simulink library "SimscapeCustomComponents_lib"  (R2025b)
settings: Solver=VariableStepAuto  StartTime=0.0  StopTime=10.0  RelTol=1e-3
undefined symbols (not defined in the file or in its folder): base, baseVdc, capacity, DiscIntNeverNeededParam, ee_sli_rtmsupport, filterInductance, freqeuncy, frequency, gcbh, gflInverter, gfmInverter, iMaxPU, Inertia, initialSOC, plantRating, solar, Ts, ups, Vac, windSystem, windTurbine
libraries: fl_lib x397, nesl_utility x171, eeGeneralControl x85, ee_lib x82, simulink x72, datacenter_lib x68, eeTransforms x38, slpidlib x24, buildingEnergy_lib x20, SimscapeFluids_lib x17, eeSinusoidalMeasurementV2 x8, eePwmGenerator x8
(part 14 of 24)

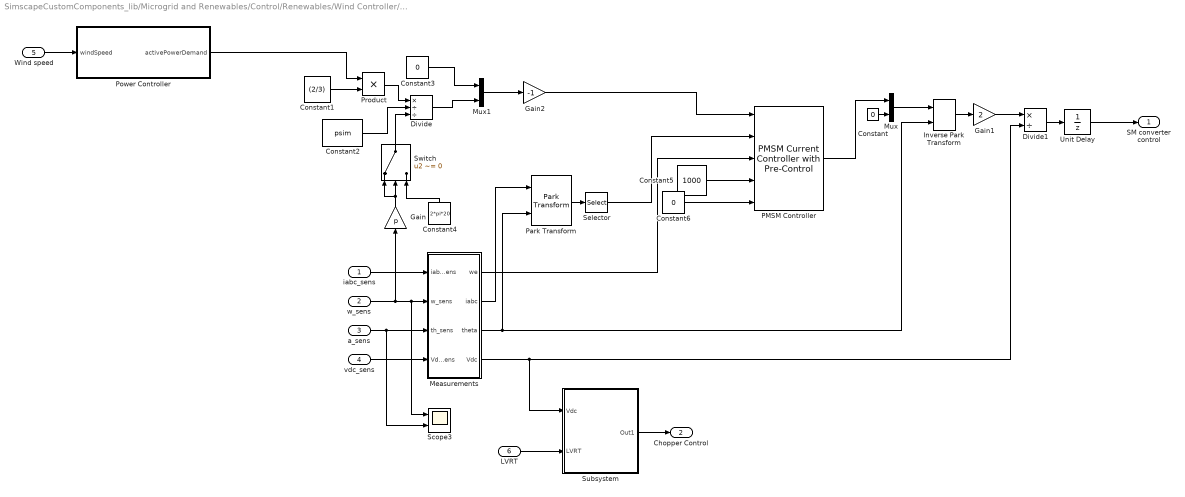
== system SimscapeCustomComponents_lib/Microgrid and Renewables/Control/Renewables/Wind Controller/Machine Converter Control ==
  iabc_sens : Inport
  w_sens : Inport  Port=2
  a_sens : Inport  Port=3
  vdc_sens : Inport  Port=4
  Wind speed : Inport  Port=5
  LVRT : Inport  Port=6
  Constant : Constant  Value=0  SampleTime=-1
  Constant1 : Constant  Value=(2/3)
  Constant2 : Constant  Value=psim
  Constant3 : Constant  Value=0
  Constant4 : Constant  Value=2*pi*20
  Constant5 : Constant  Value=1000  VectorParams1D=off  SampleTime=-1
  Constant6 : Constant  Value=0
  Divide : Product  Inputs=*//
  Divide1 : Product  Inputs=*/
  Gain : Gain  Gain=p
  Gain1 : Gain  Gain=2
  Gain2 : Gain  Gain=-1
  Inverse Park Transform : eeTransforms/Inverse Park Transform  AxisAlignment=Q-axis  PowerInvariant=off
  Measurements : Subsystem
  Mux : Mux  Inputs=2
  Mux1 : Mux  Inputs=2
  PMSM Controller : eePmsmCurrentController/PMSM Current Controller with Pre-Control  Kp_id=Kdip_sm  Ki_id=Kdii_sm  Kaw_id=0  Kp_iq=Kqip_sm  Ki_iq=Kqii_sm  Kaw_iq=0  Ts=-1  Tsd=0.001  AxisPrio=Q-axis  ActZC=off  ActFF=on  idVect=[-1, 0, 1]  iqVect=[-2000, 0, 2000]  LdMatrix=Ld* ones(3, 3)  LqMatrix=Lq* ones(3, 3)  psimMatrix=psim * ones(3, 3)
  Park Transform : eeTransforms/Park Transform  AxisAlignment=Q-axis  PowerInvariant=off
  Power Controller : Subsystem
  Product : Product
  Scope3 : Scope  NumInputPorts=2
      settings: ActiveDisplayYMinimum=-0.53154558960654574  ActiveDisplayYMaximum=3.2068078785969831  DataLoggingVariableName=ScopeData23
  Selector : Selector  InputPortWidth=3  IndexOptions=Index vector (dialog)  Indices=[1 2]  OutputSizes=1
  Subsystem : Subsystem
  Switch : Switch  Criteria=u2 ~= 0  SaturateOnIntegerOverflow=off  InputSameDT=off
  Unit Delay : UnitDelay  SampleTime=-1
  SM converter control : Outport  VectorParamsAs1DForOutWhenUnconnected=off
  Chopper Control : Outport  Port=2
  wires:
  Product/1 -> Divide/1
  Measurements/1(we) -> PMSM Controller/3
  Unit Delay/1 -> SM converter control/1
  Wind speed/1 -> Power Controller/1(windSpeed)
  Selector/1 -> PMSM Controller/2
  LVRT/1 -> Subsystem/2(LVRT)
  Divide/1 -> Mux1/2
  Constant4/1 -> Switch/3
  Gain1/1 -> Divide1/1
  PMSM Controller/1 -> Mux/1
  Mux1/1 -> Gain2/1
  Power Controller/1(activePowerDemand) -> Product/1
  Divide1/1 -> Unit Delay/1
  Constant2/1 -> Divide/2
  Constant1/1 -> Product/2
  Park Transform/1 -> Selector/1
  iabc_sens/1 -> Measurements/1(iabc_sens)
  Constant/1 -> Mux/2
  Measurements/2(iabc) -> Park Transform/1
  Constant6/1 -> PMSM Controller/5
  Switch/1 -> Divide/3
  Inverse Park Transform/1 -> Gain1/1
  Mux/1 -> Inverse Park Transform/1
  Gain2/1 -> PMSM Controller/1
  Measurements/4(Vdc) -> Subsystem/1(Vdc), Divide1/2
  vdc_sens/1 -> Measurements/4(Vdc_sens)
  Constant5/1 -> PMSM Controller/4
  Subsystem/1(Out1) -> Chopper Control/1
  Gain/1 -> Switch/1, Switch/2
  Constant3/1 -> Mux1/1
  a_sens/1 -> Scope3/2, Measurements/3(th_sens)
  w_sens/1 -> Gain/1, Scope3/1, Measurements/2(w_sens)
  Measurements/3(theta) -> Park Transform/2, Inverse Park Transform/2

== system SimscapeCustomComponents_lib/Microgrid and Renewables/Control/Renewables/Wind Controller/Wind Grid-side Converter Controller ==
  QRef : Inport
  BusElementIn : Inport  Port=2  PortName=VIBus  Element=Vmag
  BusElementIn4 : Inport  Port=2  PortName=VIBus  Element=Vmag
  BusElementIn1 : Inport  Port=2  PortName=VIBus  Element=Iabc
  BusElementIn2 : Inport  Port=2  PortName=VIBus  Element=Vq
  BusElementIn3 : Inport  Port=2  PortName=VIBus  Element=Vd
  BusElementIn5 : Inport  Port=2  PortName=VIBus  Element=Theta
  BusElementIn6 : Inport  Port=2  PortName=VIBus  Element=Theta
  LVRT : Inport  Port=3
  Vdc : Inport  Port=4
  Constant : Constant  Value=Vdc
  Current_controller : Subsystem
  "DC Bus Chopper control " : Subsystem
  DC voltage controller & current reference : Subsystem
  Demux : Demux  Outputs=3
  Inverse Park Transform1 : eeTransforms/Inverse Park Transform  AxisAlignment=Q-axis  PowerInvariant=off
  Park Transform1 : eeTransforms/Park Transform  AxisAlignment=Q-axis  PowerInvariant=off
  Terminator : Terminator
  Unit Delay2 : UnitDelay  SampleTime=Ts
  FRT : Outport
  m_abc : Outport  Port=2
  wires:
  BusElementIn3/1 -> Current_controller/5(Vd)
  BusElementIn1/1 -> Park Transform1/1
  DC voltage controller & current reference/2(iq_ref) -> Current_controller/4(iqref)
  DC voltage controller & current reference/1(id_ref) -> Current_controller/3(id-ref)
  Demux/2 -> Current_controller/2(iq)
  Demux/1 -> Current_controller/1(iWindd)
  Park Transform1/1 -> Demux/1
  BusElementIn2/1 -> Current_controller/6(Vq)
  Inverse Park Transform1/1 -> Unit Delay2/1
  Unit Delay2/1 -> m_abc/1
  Current_controller/1(Refrence_mdq0) -> Inverse Park Transform1/1
  BusElementIn6/1 -> Park Transform1/2
  BusElementIn5/1 -> Inverse Park Transform1/2
  BusElementIn4/1 -> DC voltage controller & current reference/2(Vmag)
  LVRT/1 -> DC voltage controller & current reference/5(lvrt.iq)
  QRef/1 -> DC voltage controller & current reference/1(Q_ref)
  BusElementIn/1 -> "DC Bus Chopper control "/1(In1)
  "DC Bus Chopper control "/1(Out1) -> FRT/1
  Demux/3 -> Terminator/1
  Vdc/1 -> DC voltage controller & current reference/3(Wind_Mpp_vdc)
  Constant/1 -> DC voltage controller & current reference/4(Wind_vdc)

== system SimscapeCustomComponents_lib/Microgrid and Renewables/Sources/Generator Integrated/Detailed/AVR and Exciter ==
  AVR : eeSmDC2C/SM DC2C  E_FD0=1.01  Ts=-1  R_C=0  X_C=0  T_R=0  K_A=300  T_A=0.06  T_B=0  T_C=0  K_F=0.058  T_F=0.62  V_Rmax=4.5  V_Rmin=-4.5  oelInputLocation=Unused  uelInputLocation=Unused  sclInputLocation=Unused  K_E=1  T_E=1.33  E_FDmin=-99  E_1=3.05  S_E_E1=0.279  E_2=2.29  S_E_E2=0.117
  Constant{3,5..9} (6 alike) : Constant  Value=0
  Constant4 : Constant  Value=1.05
  "E_FD Simulink-PS " : nesl_utility/Simulink-PS Converter  PhysicalDomain=network_engine_domain  SubClassName=ps_input  LeftPortType=input  RightPortType=output  PseudoPeriodic=off  Frequencies=[]  NoiseDistribution=none  NoiseParameters=[]  Unit=1  AffineConversion=off  FilteringAndDerivatives=provide  SimscapeFilterOrder=1  InputFilterTimeConstant=.001  UdotUserProvided=0
  Exciter : ee_lib/Electromechanical/Synchronous/Synchronous Machine Field Circuit  unit_option=ee.enum.unit.pu  SRated=genRating*1000 V*A  FRated=frequency Hz  fieldCircuitParameterization_option=ee.enum.sm.fieldparameterization.current  baseEfd=200 V  baseIfd=100 A  parameterization_option=2  Ladu=1.66  Rfd=0.0006  Xl=0.01  Xd=0.344  Xdd=0.026  Xddd=0.018  d_option=ee.enum.circuit.short  Td0d=machine.tauDAxisTransient s  Tdd=0.03 s  Td0dd=machine.tauDAxisSubTransient s  Tddd=0.008 s
      settings: InternalSimscapePortConfiguration="{\"Bottom\":[],\"Left\":[{\"id\":\"Efd_pu\",\"label\":\"Efd_pu\",\"type\":\"input\"},{\"id\":\"Ifd_pu\",\"label\":\"Ifd_pu\",\"type\":\"output\"}],\"Right\":[{\"id\":\"fd_p\",\"label\":\"fd+\",\"type\":\"foundation.electrical.electrical\"},{\"id\":\"fd_n\",\"label\":\"fd-\",\"type\":\"foundation.electrical.electrical\"}],\"Top\":[]}"
  I_FD PS-Simulink : nesl_utility/PS-Simulink Converter  PhysicalDomain=network_engine_domain  SubClassName=ps_output  LeftPortType=input  RightPortType=output  PseudoPeriodic=off  Frequencies=[]  VectorFormat=1-D array  Unit=1  AffineConversion=off
  Terminal Current Measurement : ee_lib/Electromechanical/Synchronous/Synchronous Machine Measurement  output_idx=15
      settings: InternalSimscapePortConfiguration="{\"Bottom\":[],\"Left\":[{\"id\":\"pu_input\",\"label\":\"pu\",\"type\":\"input\"}],\"Right\":[{\"id\":\"pu_output\",\"label\":\"o\",\"type\":\"output\"}],\"Top\":[]}"
  Terminal Current PS-Simulink : nesl_utility/PS-Simulink Converter  PhysicalDomain=network_engine_domain  SubClassName=ps_output  LeftPortType=input  RightPortType=output  PseudoPeriodic=off  Frequencies=[]  VectorFormat=1-D array  Unit=1  AffineConversion=off
  Terminal Voltage Measurement : ee_lib/Electromechanical/Synchronous/Synchronous Machine Measurement  output_idx=14
      settings: InternalSimscapePortConfiguration="{\"Bottom\":[],\"Left\":[{\"id\":\"pu_input\",\"label\":\"pu\",\"type\":\"input\"}],\"Right\":[{\"id\":\"pu_output\",\"label\":\"o\",\"type\":\"output\"}],\"Top\":[]}"
  Terminal Voltage PS-Simulink : nesl_utility/PS-Simulink Converter  PhysicalDomain=network_engine_domain  SubClassName=ps_output  LeftPortType=input  RightPortType=output  PseudoPeriodic=off  Frequencies=[]  VectorFormat=1-D array  Unit=1  AffineConversion=off
  Terminator : Terminator
  Unit Delay : UnitDelay  InitialCondition=1.32943  SampleTime=-1
  pu : PMIOPort  Side=Left
  fd+ : PMIOPort  Port=2  Side=Right
  fd- : PMIOPort  Port=3  Side=Right
  wires:
  Terminal Current PS-Simulink/1 -> AVR/4
  AVR/1 -> "E_FD Simulink-PS "/1
  Constant9/1 -> AVR/9
  Constant8/1 -> AVR/8
  Constant7/1 -> AVR/7
  Constant6/1 -> AVR/6
  Constant5/1 -> AVR/5
  Constant4/1 -> AVR/1
  Constant3/1 -> AVR/2
  Terminal Voltage PS-Simulink/1 -> AVR/3
  I_FD PS-Simulink/1 -> Unit Delay/1
  Unit Delay/1 -> Terminator/1
  connections:
  Terminal Current Measurement/RConn1 -- Terminal Current PS-Simulink/LConn1
  Terminal Voltage Measurement/RConn1 -- Terminal Voltage PS-Simulink/LConn1
  pu/RConn1 -- Terminal Current Measurement/LConn1 -- Terminal Voltage Measurement/LConn1
  Exciter/RConn1 -- fd+/RConn1
  fd-/RConn1 -- Exciter/RConn2
  I_FD PS-Simulink/LConn1 -- Exciter/LConn2
  "E_FD Simulink-PS "/RConn1 -- Exciter/LConn1

== system SimscapeCustomComponents_lib/Microgrid and Renewables/Sources/Generator Integrated/Detailed/Governor and Prime Mover  ==
  PRef : Inport
  Governor : Subsystem
  Ideal Torque Source : fl_lib/Mechanical/Mechanical Sources/Ideal Torque Source
  Mechanical Rotational Reference : fl_lib/Mechanical/Rotational Elements/Mechanical Rotational Reference
  Non-reheat turbine : Subsystem
  PS-Simulink Converter : nesl_utility/PS-Simulink Converter  PhysicalDomain=network_engine_domain  SubClassName=ps_output  LeftPortType=input  RightPortType=output  PseudoPeriodic=off  Frequencies=[]  VectorFormat=1-D array  Unit=1  AffineConversion=off
  Rotor Velocity Measurement : ee_lib/Electromechanical/Synchronous/Synchronous Machine Measurement  output_idx=4
      settings: InternalSimscapePortConfiguration="{\"Bottom\":[],\"Left\":[{\"id\":\"pu_input\",\"label\":\"pu\",\"type\":\"input\"}],\"Right\":[{\"id\":\"pu_output\",\"label\":\"o\",\"type\":\"output\"}],\"Top\":[]}"
  Scope : Scope
  Simulink-PS Converter : nesl_utility/Simulink-PS Converter  PhysicalDomain=network_engine_domain  SubClassName=ps_input  LeftPortType=input  RightPortType=output  PseudoPeriodic=off  Frequencies=[]  NoiseDistribution=none  NoiseParameters=[]  Unit=1  AffineConversion=off  FilteringAndDerivatives=zero  SimscapeFilterOrder=1  InputFilterTimeConstant=0.001  UdotUserProvided=1
  scale by base_torque : Gain  Gain=base_torque
  R : PMIOPort  Side=Right
  C : PMIOPort  Port=2  Side=Right
  pu : PMIOPort  Port=3  Side=Left
  wires:
  PS-Simulink Converter/1 -> Governor/1(pu_velocity)
  Governor/1(delta_y) -> Non-reheat turbine/1(delta_y)
  Non-reheat turbine/1(torque) -> Scope/1, scale by base_torque/1
  scale by base_torque/1 -> Simulink-PS Converter/1
  PRef/1 -> Governor/2(PRef)
  connections:
  C/RConn1 -- Ideal Torque Source/RConn2 -- Mechanical Rotational Reference/LConn1
  Ideal Torque Source/LConn1 -- R/RConn1
  pu/RConn1 -- Rotor Velocity Measurement/LConn1
  PS-Simulink Converter/LConn1 -- Rotor Velocity Measurement/RConn1
  Simulink-PS Converter/RConn1 -- Ideal Torque Source/RConn1

== system SimscapeCustomComponents_lib/Microgrid and Renewables/Sources/Generator Integrated/Detailed/Measurements ==
  Current and Voltage Sensor (Three-Phase) : ee_lib/Sensors & Transducers/Current and Voltage Sensor (Three-Phase)  vMeasurementType=ee.enum.vmeasurement.ll  outputUnit=ee.enum.unit.pu  SRated=genRating*1000 A*V  VRated=Vac V  I_specify=off  I_priority=None  I=[0, 0, 0] A  I_nominal_specify=off  I_nominal_value=1  I_nominal_unit=A  V_specify=off  V_priority=None  V=[0, 0, 0] V  V_nominal_specify=off  V_nominal_value=1  V_nominal_unit=V
      settings: InternalSimscapePortConfiguration="{\"Bottom\":[],\"Left\":[{\"id\":\"N1\",\"label\":\"~1\",\"type\":\"foundation.electrical.three_phase\"}],\"Right\":[{\"id\":\"V_output\",\"label\":\"V\",\"type\":\"output\"},{\"id\":\"I_output\",\"label\":\"I\",\"type\":\"output\"},{\"id\":\"N2\",\"label\":\"~2\",\"type\":\"foundation.electrical.three_phase\"}],\"Top\":[]}"
  Gain : Gain  Gain=1/(genRating*1000)
  Gain1 : Gain  Gain=1/(genRating*1000)
  Low-Pass Filter (Discrete or Continuous)1 : eeGeneralControl/Low-Pass Filter (Discrete or Continuous)  K=1  T=0.1  B=inf  A=-inf  init_option=Inherited from block input  x0=0  Ts=-1
  Low-Pass Filter (Discrete or Continuous)2 : eeGeneralControl/Low-Pass Filter (Discrete or Continuous)  K=1  T=0.1  B=inf  A=-inf  init_option=Inherited from block input  x0=0  Ts=-1
  PS-Simulink Converter{,1..3} (4 alike) : nesl_utility/PS-Simulink Converter  PhysicalDomain=network_engine_domain  SubClassName=ps_output  LeftPortType=input  RightPortType=output  PseudoPeriodic=off  Frequencies=[]  VectorFormat=inherit  Unit=inherit  AffineConversion=off
  Power Sensor (Three-Phase) : ee_lib/Sensors & Transducers/Power Sensor (Three-Phase)  load_type=ee.enum.passive.type_balanced.balanced  f0=60 Hz
      settings: InternalSimscapePortConfiguration="{\"Bottom\":[],\"Left\":[{\"id\":\"N1\",\"label\":\"~1\",\"type\":\"foundation.electrical.three_phase\"}],\"Right\":[{\"id\":\"N2\",\"label\":\"~2\",\"type\":\"foundation.electrical.three_phase\"}],\"Top\":[{\"id\":\"Pm\",\"label\":\"P\",\"type\":\"output\"},{\"id\":\"Qm\",\"label\":\"Q\",\"type\":\"output\"}]}"
  In : PMIOPort  Side=Left
  ~ : PMIOPort  Port=2  Side=Right
  P : Outport
  Q : Outport  Port=2
  V : Outport  Port=3
  I : Outport  Port=4
  wires:
  PS-Simulink Converter/1 -> Low-Pass Filter (Discrete or Continuous)1/1
  PS-Simulink Converter1/1 -> Low-Pass Filter (Discrete or Continuous)2/1
  Low-Pass Filter (Discrete or Continuous)1/1 -> Gain/1
  Low-Pass Filter (Discrete or Continuous)2/1 -> Gain1/1
  PS-Simulink Converter2/1 -> V/1
  PS-Simulink Converter3/1 -> I/1
  Gain/1 -> P/1
  Gain1/1 -> Q/1
  connections:
  Current and Voltage Sensor (Three-Phase)/RConn1 -- PS-Simulink Converter2/LConn1
  PS-Simulink Converter/LConn1 -- Power Sensor (Three-Phase)/LConn2
  In/RConn1 -- Power Sensor (Three-Phase)/LConn1
  Current and Voltage Sensor (Three-Phase)/RConn3 -- ~/RConn1
  PS-Simulink Converter1/LConn1 -- Power Sensor (Three-Phase)/LConn3
  Current and Voltage Sensor (Three-Phase)/LConn1 -- Power Sensor (Three-Phase)/RConn1
  Current and Voltage Sensor (Three-Phase)/RConn2 -- PS-Simulink Converter3/LConn1

== system SimscapeCustomComponents_lib/Microgrid and Renewables/Sources/Generator Integrated/Simplified/Exciter ==
  Current Sensor : fl_lib/Electrical/Electrical Sensors/Current Sensor
  Voltage Source : ee_lib/Sources/Voltage Source  dc_voltage=150 V  ac_voltage=0 V  ac_shift=0 rad  ac_frequency=frequency Hz  noise_mode=ee.enum.sources.noise.Disabled  PSD=0 V^2/Hz  sample_time=1e-3 s  repeatability=ee.enum.sources.repeatability.NotRepeatable  user_seed=0  auto_seed=3890346746  i_specify=off  i_priority=None  i=0 A  i_nominal_specify=off  i_nominal_value=1  i_nominal_unit=A  v_specify=off  v_priority=None  v=0 V  v_nominal_specify=off  v_nominal_value=1  v_nominal_unit=V
  + : PMIOPort  Side=Right
  - : PMIOPort  Port=2  Side=Right
  connections:
  Voltage Source/RConn1 -- -/RConn1
  Current Sensor/RConn2 -- +/RConn1
  Voltage Source/LConn1 -- Current Sensor/LConn1

== system SimscapeCustomComponents_lib/Microgrid and Renewables/Sources/Generator Integrated/Simplified/Measurements ==
  Current and Voltage Sensor (Three-Phase) : ee_lib/Sensors & Transducers/Current and Voltage Sensor (Three-Phase)  vMeasurementType=ee.enum.vmeasurement.ll  outputUnit=ee.enum.unit.pu  SRated=genRating*1000 A*V  VRated=Vac V  I_specify=off  I_priority=None  I=[0, 0, 0] A  I_nominal_specify=off  I_nominal_value=1  I_nominal_unit=A  V_specify=off  V_priority=None  V=[0, 0, 0] V  V_nominal_specify=off  V_nominal_value=1  V_nominal_unit=V
      settings: InternalSimscapePortConfiguration="{\"Bottom\":[],\"Left\":[{\"id\":\"N1\",\"label\":\"~1\",\"type\":\"foundation.electrical.three_phase\"}],\"Right\":[{\"id\":\"V_output\",\"label\":\"V\",\"type\":\"output\"},{\"id\":\"I_output\",\"label\":\"I\",\"type\":\"output\"},{\"id\":\"N2\",\"label\":\"~2\",\"type\":\"foundation.electrical.three_phase\"}],\"Top\":[]}"
  Gain : Gain  Gain=1/(genRating*1000)
  Gain1 : Gain  Gain=1/(genRating*1000)
  Low-Pass Filter (Discrete or Continuous)1 : eeGeneralControl/Low-Pass Filter (Discrete or Continuous)  K=1  T=0.1  B=inf  A=-inf  init_option=Inherited from block input  x0=0  Ts=-1
  Low-Pass Filter (Discrete or Continuous)2 : eeGeneralControl/Low-Pass Filter (Discrete or Continuous)  K=1  T=0.1  B=inf  A=-inf  init_option=Inherited from block input  x0=0  Ts=-1
  PS-Simulink Converter{,1..3} (4 alike) : nesl_utility/PS-Simulink Converter  PhysicalDomain=network_engine_domain  SubClassName=ps_output  LeftPortType=input  RightPortType=output  PseudoPeriodic=off  Frequencies=[]  VectorFormat=inherit  Unit=inherit  AffineConversion=off
  Power Sensor (Three-Phase) : ee_lib/Sensors & Transducers/Power Sensor (Three-Phase)  load_type=ee.enum.passive.type_balanced.balanced  f0=60 Hz
      settings: InternalSimscapePortConfiguration="{\"Bottom\":[],\"Left\":[{\"id\":\"N1\",\"label\":\"~1\",\"type\":\"foundation.electrical.three_phase\"}],\"Right\":[{\"id\":\"N2\",\"label\":\"~2\",\"type\":\"foundation.electrical.three_phase\"}],\"Top\":[{\"id\":\"Pm\",\"label\":\"P\",\"type\":\"output\"},{\"id\":\"Qm\",\"label\":\"Q\",\"type\":\"output\"}]}"
  In : PMIOPort  Side=Left
  ~ : PMIOPort  Port=2  Side=Right
  P : Outport
  Q : Outport  Port=2
  V : Outport  Port=3
  I : Outport  Port=4
  wires:
  PS-Simulink Converter/1 -> Low-Pass Filter (Discrete or Continuous)1/1
  PS-Simulink Converter1/1 -> Low-Pass Filter (Discrete or Continuous)2/1
  Low-Pass Filter (Discrete or Continuous)1/1 -> Gain/1
  Low-Pass Filter (Discrete or Continuous)2/1 -> Gain1/1
  PS-Simulink Converter2/1 -> V/1
  PS-Simulink Converter3/1 -> I/1
  Gain/1 -> P/1
  Gain1/1 -> Q/1
  connections:
  Current and Voltage Sensor (Three-Phase)/RConn1 -- PS-Simulink Converter2/LConn1
  PS-Simulink Converter/LConn1 -- Power Sensor (Three-Phase)/LConn2
  In/RConn1 -- Power Sensor (Three-Phase)/LConn1
  Current and Voltage Sensor (Three-Phase)/RConn3 -- ~/RConn1
  PS-Simulink Converter1/LConn1 -- Power Sensor (Three-Phase)/LConn3
  Current and Voltage Sensor (Three-Phase)/LConn1 -- Power Sensor (Three-Phase)/RConn1
  Current and Voltage Sensor (Three-Phase)/RConn2 -- PS-Simulink Converter3/LConn1

== system SimscapeCustomComponents_lib/Microgrid and Renewables/Sources/Generator Integrated/Simplified/Prime Mover ==
  PRef : Inport
  Ideal Torque Source : fl_lib/Mechanical/Mechanical Sources/Ideal Torque Source
  Mechanical Rotational Reference : fl_lib/Mechanical/Rotational Elements/Mechanical Rotational Reference
  Saturation : Saturate  UpperLimit=1  LowerLimit=0
  Scope : Scope
      settings: ActiveDisplayYMinimum=-1.25  ActiveDisplayYMaximum=1.25
  Simulink-PS Converter : nesl_utility/Simulink-PS Converter  PhysicalDomain=network_engine_domain  SubClassName=ps_input  LeftPortType=input  RightPortType=output  PseudoPeriodic=off  Frequencies=[]  NoiseDistribution=none  NoiseParameters=[]  Unit=1  AffineConversion=off  FilteringAndDerivatives=zero  SimscapeFilterOrder=1  InputFilterTimeConstant=0.001  UdotUserProvided=1
  scale by base_torque : Gain  Gain=genRating*1000/(2*pi*frequency)
  R : PMIOPort  Side=Right
  C : PMIOPort  Port=2  Side=Right
  wires:
  PRef/1 -> Saturation/1, Scope/1
  scale by base_torque/1 -> Simulink-PS Converter/1
  Saturation/1 -> scale by base_torque/1
  connections:
  Ideal Torque Source/LConn1 -- R/RConn1
  C/RConn1 -- Mechanical Rotational Reference/LConn1 -- Ideal Torque Source/RConn2
  Simulink-PS Converter/RConn1 -- Ideal Torque Source/RConn1

== system SimscapeCustomComponents_lib/Microgrid and Renewables/Sources/Solar Plant/Converter/Average ==
  mabc : Inport
  Converter : ee_lib/Semiconductors & Converters/Converters/Average-Value Voltage Source Converter (Three-Phase)  port_option=ee.enum.threePhasePort.composite  frequency_option=ee.enum.converters.frequency.variable  input_option=ee.enum.converters.inputOption.ModWave  FRated=60 Hz  losses_parameterization=ee.enum.converters.losses.fixed  Pfixed=0.5 W  ks=0.01  kc1=1.7 V  kc2=0.01 Ohm  Ploss_vect=[100, 800, 1870, 3250, 4900] W  Irms_vect=[10, 100, 200, 300, 400] A  Vdc_nom=300 V  thermal_mass=30000 J/K  temperature_specify=off  temperature_priority=High  temperature=298.15 K  temperature_nominal_specify=off  temperature_nominal_value=1  temperature_nominal_unit=K
      settings: InternalSimscapePortConfiguration="{\"Bottom\":[],\"Left\":[{\"id\":\"ModWave\",\"label\":\"ModWave\",\"type\":\"input\"},{\"id\":\"N\",\"label\":\"~\",\"type\":\"foundation.electrical.three_phase\"}],\"Right\":[{\"id\":\"p\",\"label\":\"+\",\"type\":\"foundation.electrical.electrical\"},{\"id\":\"n\",\"label\":\"-\",\"type\":\"foundation.electrical.electrical\"}],\"Top\":[]}"
  Simulink-PS Converter : nesl_utility/Simulink-PS Converter  PhysicalDomain=network_engine_domain  SubClassName=ps_input  LeftPortType=input  RightPortType=output  PseudoPeriodic=off  Frequencies=[]  NoiseDistribution=none  NoiseParameters=[]  Unit=1  AffineConversion=off  FilteringAndDerivatives=provide  SimscapeFilterOrder=1  InputFilterTimeConstant=0.001  UdotUserProvided=0
  + : PMIOPort  Side=Left
  - : PMIOPort  Port=2  Side=Left
  ~ : PMIOPort  Port=3  Side=Right
  wires:
  mabc/1 -> Simulink-PS Converter/1
  connections:
  +/RConn1 -- Converter/RConn1
  -/RConn1 -- Converter/RConn2
  ~/RConn1 -- Converter/LConn2
  Simulink-PS Converter/RConn1 -- Converter/LConn1

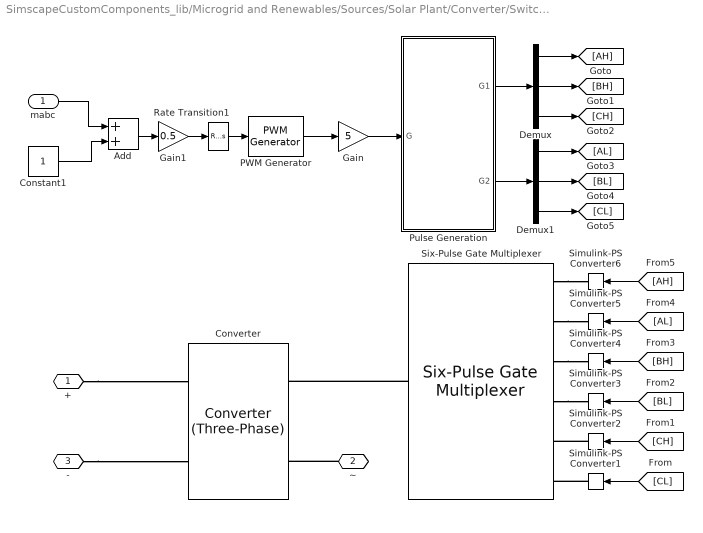
== system SimscapeCustomComponents_lib/Microgrid and Renewables/Sources/Solar Plant/Converter/Switching ==
  mabc : Inport
  Add : Sum
  Constant1 : Constant
  Converter : ee_lib/Semiconductors & Converters/Converters/Converter (Three-Phase)  port_option=ee.enum.threePhasePort.composite  fidelity_option=ee.enum.converters.fidelity.detailed  device_type=ee.enum.converters.switchingdevice.ideal  showThermalPort=false  K=0  Vth=1 V  Vgt=1 V  Vgt_off=-1 V  Ih=1 A  Vf=0.8 V  Ron=0.001 Ohm  Rds=0.001 Ohm  Goff=1e-6 1/Ohm  Eon_scalar=22.86e-3 J  Eoff_scalar=17.14e-3 J  Eoff_natural_commutation=10e-3 J  Voff=300 V  Iout_scalar=600 A  onCurrentMeasDelay=0 s  useCurrentFromPreviousCycle=false  useVoltageFromPreviousCycle=false  diode_param=ee.enum.converters.protectiondiode.nodynamics  diode_Vf=0.01 V  diode_Ron=0.0001 Ohm  diode_Goff=1e-5 1/Ohm  diode_C=50 nF  diode_iRM=-235 A  diode_iF=300 A  diode_idot=-50 A/us  diode_trr_param=ee.enum.converters.diodetrr.trr_factor  diode_trr_factor=3  diode_trr=15 us  diode_Qrr=1500 s*uA  diode_rec_loss_model=ee.enum.diode.reverseRecoveryModel.fixed  diode_ErecVal=0 J  diode_scaleWithIandV=false  diode_ErecMat=zeros(2, 3) J  diode_TjrecVec=[298.15, 398.15] K  diode_IfrecVec=[.1, 1, 10] A  diode_IrecVal=10 A  diode_VrecVal=10 V  diode_tFilter=1 / 1000 / 100 s  thermal_network_parameterization=ee.enum.thermalNetworkTopology.external  Rth=[.08, .5] K/W  Rth_Cauer=[.08, .1, .5] K/W  Rth_Foster=[.08, .14, .22, .16] K/W  thermal_mass_parameterization=ee.enum.thermalNetwork.timeconstant  thermal_mass=[.01, .5] J/K  thermal_mass_Cauer=[.01, .1, .5] J/K  thermal_mass_Foster=[.001, .005, .05, .5] J/K  thermal_time_constant=[.001, .2] s  thermal_time_constant_Cauer=[.001, .1, .2] s  thermal_time_constant_Foster=[7e-05, .0007, .01, .08] s  thermal_mass_initial_temperatures=[25, 25] degC  thermal_mass_initial_temperatures_Cauer=[25, 25, 25] degC  junction_thermal_mass=0.01 J/K  Tvec_initial_Foster=[25, 25, 25, 25] degC  snubber_type=ee.enum.converters.snubber.exclude  Cs=1e-7 F  Rs=0.1 Ohm  Vce_loss=[0, 150, 300] V
  Demux : Demux  Outputs=3
  Demux1 : Demux  Outputs=3
  Gain : Gain  Gain=5
  Gain1 : Gain  Gain=0.5
  PWM Generator : eePwmGenerator/PWM Generator  CarrCount=Up  Tper=1/(fSw*1000)  Tdelay=0  Ts=1/(10*fSw*1000)
  Pulse Generation : Subsystem
  Rate Transition1 : RateTransition  OutPortSampleTime=1/(10*fSw*1000)
  Simulink-PS Converter{1..6} (6 alike) : nesl_utility/Simulink-PS Converter  PhysicalDomain=network_engine_domain  SubClassName=ps_input  LeftPortType=input  RightPortType=output  PseudoPeriodic=off  Frequencies=[]  NoiseDistribution=none  NoiseParameters=[]  Unit=1  AffineConversion=off  FilteringAndDerivatives=provide  SimscapeFilterOrder=1  InputFilterTimeConstant=0.001  UdotUserProvided=0
  Six-Pulse Gate Multiplexer : ee_lib/Semiconductors & Converters/Converters/Six-Pulse Gate Multiplexer  port_option=ee.enum.controlport.ps
  + : PMIOPort  Side=Left
  ~ : PMIOPort  Port=2  Side=Right
  - : PMIOPort  Port=3  Side=Left
  wires:
  [BH] -> Simulink-PS Converter4/1
  Pulse Generation/1(G1) -> Demux/1
  Pulse Generation/2(G2) -> Demux1/1
  Rate Transition1/1 -> PWM Generator/1
  Demux/1 -> [AH]
  Demux1/2 -> [BL]
  [AL] -> Simulink-PS Converter5/1
  [CH] -> Simulink-PS Converter2/1
  mabc/1 -> Add/1
  PWM Generator/1 -> Gain/1
  Gain/1 -> Pulse Generation/1(G)
  Add/1 -> Gain1/1
  Constant1/1 -> Add/2
  [CL] -> Simulink-PS Converter1/1
  Demux/2 -> [BH]
  Demux/3 -> [CH]
  Gain1/1 -> Rate Transition1/1
  Demux1/3 -> [CL]
  [AH] -> Simulink-PS Converter6/1
  [BL] -> Simulink-PS Converter3/1
  Demux1/1 -> [AL]
  connections:
  -/RConn1 -- Converter/RConn2
  +/RConn1 -- Converter/RConn1
  Six-Pulse Gate Multiplexer/LConn4 -- Simulink-PS Converter3/RConn1
  Six-Pulse Gate Multiplexer/LConn1 -- Simulink-PS Converter6/RConn1
  Six-Pulse Gate Multiplexer/RConn1 -- Converter/LConn1
  Six-Pulse Gate Multiplexer/LConn3 -- Simulink-PS Converter4/RConn1
  Simulink-PS Converter1/RConn1 -- Six-Pulse Gate Multiplexer/LConn6
  Simulink-PS Converter2/RConn1 -- Six-Pulse Gate Multiplexer/LConn5
  Six-Pulse Gate Multiplexer/LConn2 -- Simulink-PS Converter5/RConn1
  ~/RConn1 -- Converter/LConn2

== system SimscapeCustomComponents_lib/Microgrid and Renewables/Sources/Solar Plant Integrated/Detailed/Measurements ==
  Current and Voltage Sensor (Three-Phase) : ee_lib/Sensors & Transducers/Current and Voltage Sensor (Three-Phase)  vMeasurementType=ee.enum.vmeasurement.lg  outputUnit=ee.enum.unit.pu  SRated=plantRating*1000 A*V  VRated=Vac V  I_specify=off  I_priority=None  I=[0, 0, 0] A  I_nominal_specify=off  I_nominal_value=1  I_nominal_unit=A  V_specify=off  V_priority=None  V=[0, 0, 0] V  V_nominal_specify=off  V_nominal_value=1  V_nominal_unit=V
      settings: InternalSimscapePortConfiguration="{\"Bottom\":[],\"Left\":[{\"id\":\"N1\",\"label\":\"~1\",\"type\":\"foundation.electrical.three_phase\"}],\"Right\":[{\"id\":\"V_output\",\"label\":\"V\",\"type\":\"output\"},{\"id\":\"I_output\",\"label\":\"I\",\"type\":\"output\"},{\"id\":\"N2\",\"label\":\"~2\",\"type\":\"foundation.electrical.three_phase\"}],\"Top\":[]}"
  Gain : Gain  Gain=1/(plantRating*1000)
  Gain1 : Gain  Gain=1/(plantRating*1000)
  Low-Pass Filter (Discrete or Continuous)1 : eeGeneralControl/Low-Pass Filter (Discrete or Continuous)  K=1  T=0.1  B=inf  A=-inf  init_option=Inherited from block input  x0=0  Ts=-1
  Low-Pass Filter (Discrete or Continuous)2 : eeGeneralControl/Low-Pass Filter (Discrete or Continuous)  K=1  T=0.1  B=inf  A=-inf  init_option=Inherited from block input  x0=0  Ts=-1
  PS-Simulink Converter{,1..3} (4 alike) : nesl_utility/PS-Simulink Converter  PhysicalDomain=network_engine_domain  SubClassName=ps_output  LeftPortType=input  RightPortType=output  PseudoPeriodic=off  Frequencies=[]  VectorFormat=inherit  Unit=inherit  AffineConversion=off
  Power Sensor (Three-Phase) : ee_lib/Sensors & Transducers/Power Sensor (Three-Phase)  load_type=ee.enum.passive.type_balanced.balanced  f0=60 Hz
      settings: InternalSimscapePortConfiguration="{\"Bottom\":[],\"Left\":[{\"id\":\"N1\",\"label\":\"~1\",\"type\":\"foundation.electrical.three_phase\"}],\"Right\":[{\"id\":\"N2\",\"label\":\"~2\",\"type\":\"foundation.electrical.three_phase\"}],\"Top\":[{\"id\":\"Pm\",\"label\":\"P\",\"type\":\"output\"},{\"id\":\"Qm\",\"label\":\"Q\",\"type\":\"output\"}]}"
  In : PMIOPort  Side=Left
  ~ : PMIOPort  Port=2  Side=Right
  P : Outport
  Q : Outport  Port=2
  V : Outport  Port=3
  I : Outport  Port=4
  wires:
  PS-Simulink Converter/1 -> Low-Pass Filter (Discrete or Continuous)1/1
  PS-Simulink Converter1/1 -> Low-Pass Filter (Discrete or Continuous)2/1
  Low-Pass Filter (Discrete or Continuous)1/1 -> Gain/1
  Low-Pass Filter (Discrete or Continuous)2/1 -> Gain1/1
  PS-Simulink Converter2/1 -> V/1
  PS-Simulink Converter3/1 -> I/1
  Gain/1 -> P/1
  Gain1/1 -> Q/1
  connections:
  Current and Voltage Sensor (Three-Phase)/RConn1 -- PS-Simulink Converter2/LConn1
  PS-Simulink Converter/LConn1 -- Power Sensor (Three-Phase)/LConn2
  In/RConn1 -- Power Sensor (Three-Phase)/LConn1
  Current and Voltage Sensor (Three-Phase)/RConn3 -- ~/RConn1
  PS-Simulink Converter1/LConn1 -- Power Sensor (Three-Phase)/LConn3
  Current and Voltage Sensor (Three-Phase)/LConn1 -- Power Sensor (Three-Phase)/RConn1
  Current and Voltage Sensor (Three-Phase)/RConn2 -- PS-Simulink Converter3/LConn1

== system SimscapeCustomComponents_lib/Microgrid and Renewables/Sources/Solar Plant Integrated/Detailed/PV Plant & Controller ==
  note: Plant
  note: Controller
  Insolation : Inport
  Pref : Inport  Port=2
  Qref : Inport  Port=3
  Vabc : Inport  Port=4
  Iabc : Inport  Port=5
  Mode : Inport  Port=6
  Controller : Subsystem
  Delay : Delay  DelayLength=1
  PV Plant : Subsystem  InitFcn=%solar.mask.restoreSolarLink(gcb);  mask(Solar Plant){capDC=capacitance, converterFidelity=Switching, fSw=fSw, ratedVoltage=Vac, nSeries=nSeries, nParallel=nParallel}
      mask prompts: capDC "DC bus capacitance (F)"; converterFidelity "Converter Fidelity"; fSw "Switching Frequency (kHz)"; ratedVoltage "Rated voltage on AC side (V)"; nSeries "Number of panels in series"; nParallel "Number of panels in parallel"
      mask help: This block represents the physical interface between the solar panels and the power converter. It models the electrical and dynamic characteristics of the solar panels connected to a converter, while expecting an external control signal for operation
      settings: CopyFcn=set_param(gcbh,'LinkStatus','none');  PreSaveFcn=%solar.mask.restoreSolarLink(gcb);  CloseFcn=%solar.mask.restoreSolarLink(gcb);
      mask TypeOptions converterFidelity: Converter/converterFidelity
      mask Callback converterFidelity: component.mask.converterFidelityPlant;
      mask TypeOptions fSw: Converter/fSw
      mask DialogControl Container4 Prompt: General
      mask DialogControl editSolarCell Prompt: Edit Solar Cell Parameters
      mask DialogControl editSolarCell Callback:
      | blockPath = [gcb,'/','PV Array'];
      | component.mask.openBlock(blockPath);;
      mask DialogControl editConverter Prompt: Edit converter parameters
      mask DialogControl editConverter Callback:
      | converterFidelity = get_param(gcb,'converterFidelity');
      | blockPath = [gcb,'/','Converter','/',converterFidelity,'/','Converter'];
      | component.mask.openBlock(blockPath);
      mask Display: image('solar1.png');
  Scope1 : Scope
      settings: ActiveDisplayYMinimum=-2.35685  ActiveDisplayYMaximum=2.29234  DataLoggingVariableName=ScopeData4
  Sensor Dynamics : Subsystem
  Simulink-PS Converter : nesl_utility/Simulink-PS Converter  PhysicalDomain=network_engine_domain  SubClassName=ps_input  LeftPortType=input  RightPortType=output  PseudoPeriodic=off  Frequencies=[]  NoiseDistribution=none  NoiseParameters=[]  Unit=1  AffineConversion=off  FilteringAndDerivatives=provide  SimscapeFilterOrder=1  InputFilterTimeConstant=0.001  UdotUserProvided=0
  abc : PMIOPort  Side=Right
  wires:
  Mode/1 -> Controller/7(Mode)
  Iabc/1 -> Controller/5(Iabc)
  Vabc/1 -> Controller/4(Vabc)
  Pref/1 -> Controller/6(Pref)
  Qref/1 -> Controller/1(Qref)
  Sensor Dynamics/1(I) -> Controller/2(ipv (A))
  Sensor Dynamics/2(V) -> Controller/3(vdc (V))
  Controller/1(vabcRef (pu)) -> Delay/1, Scope1/1
  Insolation/1 -> Simulink-PS Converter/1
  Delay/1 -> PV Plant/1(mabc)
  PV Plant/1(I) -> Sensor Dynamics/1(Iin)
  PV Plant/2(V) -> Sensor Dynamics/2(Vin)
  connections:
  PV Plant/LConn1 -- Simulink-PS Converter/RConn1
  abc/RConn1 -- PV Plant/RConn1

== system SimscapeCustomComponents_lib/Microgrid and Renewables/Sources/Solar Plant Integrated/Simplified/Measurements ==
  Current and Voltage Sensor (Three-Phase) : ee_lib/Sensors & Transducers/Current and Voltage Sensor (Three-Phase)  vMeasurementType=ee.enum.vmeasurement.lg  outputUnit=ee.enum.unit.pu  SRated=plantRating*1000 A*V  VRated=Vac V  I_specify=off  I_priority=None  I=[0, 0, 0] A  I_nominal_specify=off  I_nominal_value=1  I_nominal_unit=A  V_specify=off  V_priority=None  V=[0, 0, 0] V  V_nominal_specify=off  V_nominal_value=1  V_nominal_unit=V
      settings: InternalSimscapePortConfiguration="{\"Bottom\":[],\"Left\":[{\"id\":\"N1\",\"label\":\"~1\",\"type\":\"foundation.electrical.three_phase\"}],\"Right\":[{\"id\":\"V_output\",\"label\":\"V\",\"type\":\"output\"},{\"id\":\"I_output\",\"label\":\"I\",\"type\":\"output\"},{\"id\":\"N2\",\"label\":\"~2\",\"type\":\"foundation.electrical.three_phase\"}],\"Top\":[]}"
  Gain : Gain  Gain=1/(plantRating*1000)
  Gain1 : Gain  Gain=1/(plantRating*1000)
  Low-Pass Filter (Discrete or Continuous)1 : eeGeneralControl/Low-Pass Filter (Discrete or Continuous)  K=1  T=0.1  B=inf  A=-inf  init_option=Inherited from block input  x0=0  Ts=-1
  Low-Pass Filter (Discrete or Continuous)2 : eeGeneralControl/Low-Pass Filter (Discrete or Continuous)  K=1  T=0.1  B=inf  A=-inf  init_option=Inherited from block input  x0=0  Ts=-1
  PS-Simulink Converter{,1..3} (4 alike) : nesl_utility/PS-Simulink Converter  PhysicalDomain=network_engine_domain  SubClassName=ps_output  LeftPortType=input  RightPortType=output  PseudoPeriodic=off  Frequencies=[]  VectorFormat=inherit  Unit=inherit  AffineConversion=off
  Power Sensor (Three-Phase) : ee_lib/Sensors & Transducers/Power Sensor (Three-Phase)  load_type=ee.enum.passive.type_balanced.balanced  f0=60 Hz
      settings: InternalSimscapePortConfiguration="{\"Bottom\":[],\"Left\":[{\"id\":\"N1\",\"label\":\"~1\",\"type\":\"foundation.electrical.three_phase\"}],\"Right\":[{\"id\":\"N2\",\"label\":\"~2\",\"type\":\"foundation.electrical.three_phase\"}],\"Top\":[{\"id\":\"Pm\",\"label\":\"P\",\"type\":\"output\"},{\"id\":\"Qm\",\"label\":\"Q\",\"type\":\"output\"}]}"
  In : PMIOPort  Side=Left
  ~ : PMIOPort  Port=2  Side=Right
  P : Outport
  Q : Outport  Port=2
  V : Outport  Port=3
  I : Outport  Port=4
  wires:
  PS-Simulink Converter/1 -> Low-Pass Filter (Discrete or Continuous)1/1
  PS-Simulink Converter1/1 -> Low-Pass Filter (Discrete or Continuous)2/1
  Low-Pass Filter (Discrete or Continuous)1/1 -> Gain/1
  Low-Pass Filter (Discrete or Continuous)2/1 -> Gain1/1
  PS-Simulink Converter2/1 -> V/1
  PS-Simulink Converter3/1 -> I/1
  Gain/1 -> P/1
  Gain1/1 -> Q/1
  connections:
  Current and Voltage Sensor (Three-Phase)/RConn1 -- PS-Simulink Converter2/LConn1
  PS-Simulink Converter/LConn1 -- Power Sensor (Three-Phase)/LConn2
  In/RConn1 -- Power Sensor (Three-Phase)/LConn1
  Current and Voltage Sensor (Three-Phase)/RConn3 -- ~/RConn1
  PS-Simulink Converter1/LConn1 -- Power Sensor (Three-Phase)/LConn3
  Current and Voltage Sensor (Three-Phase)/LConn1 -- Power Sensor (Three-Phase)/RConn1
  Current and Voltage Sensor (Three-Phase)/RConn2 -- PS-Simulink Converter3/LConn1

== system SimscapeCustomComponents_lib/Microgrid and Renewables/Sources/Wind Plant/Back-to-Back Converters/Average ==
  Chopper : Inport
  SM_ref : Inport  Port=2
  Grid_ref : Inport  Port=3
  Capacitor : fl_lib/Electrical/Electrical Elements/Capacitor  c=capDC F  r=1e-1 Ohm  g=0 1/Ohm  i_specify=off  i_priority=None  i=0 A  i_nominal_specify=off  i_nominal_value=1  i_nominal_unit=A  v_specify=off  v_priority=None  v=0 V  v_nominal_specify=off  v_nominal_value=1  v_nominal_unit=V  vc_specify=on  vc_priority=High  vc=Vdc V  vc_nominal_specify=off  vc_nominal_value=1  vc_nominal_unit=V
  Electrical Reference : fl_lib/Electrical/Electrical Elements/Electrical Reference
  Electrical Reference1 : fl_lib/Electrical/Electrical Elements/Electrical Reference
  Electrical Reference2 : fl_lib/Electrical/Electrical Elements/Electrical Reference
  Grid Side Converter : ee_lib/Semiconductors & Converters/Converters/Average-Value Voltage Source Converter (Three-Phase)  port_option=ee.enum.threePhasePort.composite  frequency_option=ee.enum.converters.frequency.variable  input_option=ee.enum.converters.inputOption.ModWave  FRated=60 Hz  losses_parameterization=ee.enum.converters.losses.fixed  Pfixed=1 W  ks=0.01  kc1=1.7 V  kc2=0.01 Ohm  Ploss_vect=[100, 800, 1870, 3250, 4900] W  Irms_vect=[10, 100, 200, 300, 400] A  Vdc_nom=300 V  thermal_mass=30000 J/K  temperature_specify=off  temperature_priority=High  temperature=298.15 K  temperature_nominal_specify=off  temperature_nominal_value=1  temperature_nominal_unit=K
      settings: InternalSimscapePortConfiguration="{\"Bottom\":[],\"Left\":[{\"id\":\"ModWave\",\"label\":\"ModWave\",\"type\":\"input\"},{\"id\":\"N\",\"label\":\"~\",\"type\":\"foundation.electrical.three_phase\"}],\"Right\":[{\"id\":\"p\",\"label\":\"+\",\"type\":\"foundation.electrical.electrical\"},{\"id\":\"n\",\"label\":\"-\",\"type\":\"foundation.electrical.electrical\"}],\"Top\":[]}"
  Ideal Semiconductor Switch : ee_lib/Semiconductors & Converters/Ideal Semiconductor Switch  port_option=ee.enum.controlport.ps  Ron=0.001 Ohm  Goff=1e-6 1/Ohm  Vth=0.5 V  diode_param=ee.enum.converters.protectiondiode.none  diode_Vf=0.8 V  diode_Ron=0.001 Ohm  diode_Goff=1e-5 1/Ohm  diode_C=50e-9 F  diode_iRM=-235 A  diode_iF=300 A  diode_idot=-50 A/us  diode_trr_param=ee.enum.converters.diodetrr.trr_factor  diode_trr_factor=3  diode_trr=15 us  diode_Qrr=1500 s*uA
  Machine Side Converter : ee_lib/Semiconductors & Converters/Converters/Average-Value Voltage Source Converter (Three-Phase)  port_option=ee.enum.threePhasePort.composite  frequency_option=ee.enum.converters.frequency.variable  input_option=ee.enum.converters.inputOption.ModWave  FRated=60 Hz  losses_parameterization=ee.enum.converters.losses.fixed  Pfixed=1 W  ks=0.01  kc1=1.7 V  kc2=0.01 Ohm  Ploss_vect=[100, 800, 1870, 3250, 4900] W  Irms_vect=[10, 100, 200, 300, 400] A  Vdc_nom=300 V  thermal_mass=30000 J/K  temperature_specify=off  temperature_priority=High  temperature=298.15 K  temperature_nominal_specify=off  temperature_nominal_value=1  temperature_nominal_unit=K
      settings: InternalSimscapePortConfiguration="{\"Bottom\":[],\"Left\":[{\"id\":\"ModWave\",\"label\":\"ModWave\",\"type\":\"input\"},{\"id\":\"N\",\"label\":\"~\",\"type\":\"foundation.electrical.three_phase\"}],\"Right\":[{\"id\":\"p\",\"label\":\"+\",\"type\":\"foundation.electrical.electrical\"},{\"id\":\"n\",\"label\":\"-\",\"type\":\"foundation.electrical.electrical\"}],\"Top\":[]}"
  PS-Simulink Converter1 : nesl_utility/PS-Simulink Converter  PhysicalDomain=network_engine_domain  SubClassName=ps_output  LeftPortType=input  RightPortType=output  PseudoPeriodic=off  Frequencies=[]  VectorFormat=1-D array  Unit=V  AffineConversion=off
  Resistor : fl_lib/Electrical/Electrical Elements/Resistor  R=16 Ohm  i_specify=off  i_priority=None  i=0 A  i_nominal_specify=off  i_nominal_value=1  i_nominal_unit=A  v_specify=off  v_priority=None  v=0 V  v_nominal_specify=off  v_nominal_value=1  v_nominal_unit=V
  Scope : Scope
      settings: ActiveDisplayYMinimum=-0.125  ActiveDisplayYMaximum=1.125  DataLoggingVariableName=ScopeData11
  Simulink-PS Converter : nesl_utility/Simulink-PS Converter  PhysicalDomain=network_engine_domain  SubClassName=ps_input  LeftPortType=input  RightPortType=output  PseudoPeriodic=off  Frequencies=[]  NoiseDistribution=none  NoiseParameters=[]  Unit=1  AffineConversion=off  FilteringAndDerivatives=provide  SimscapeFilterOrder=1  InputFilterTimeConstant=0.001  UdotUserProvided=0
  Simulink-PS Converter2 : nesl_utility/Simulink-PS Converter  PhysicalDomain=network_engine_domain  SubClassName=ps_input  LeftPortType=input  RightPortType=output  PseudoPeriodic=off  Frequencies=[]  NoiseDistribution=none  NoiseParameters=[]  Unit=1  AffineConversion=off  FilteringAndDerivatives=provide  SimscapeFilterOrder=1  InputFilterTimeConstant=0.001  UdotUserProvided=0
  Simulink-PS Converter4 : nesl_utility/Simulink-PS Converter  PhysicalDomain=network_engine_domain  SubClassName=ps_input  LeftPortType=input  RightPortType=output  PseudoPeriodic=off  Frequencies=[]  NoiseDistribution=none  NoiseParameters=[]  Unit=1  AffineConversion=off  FilteringAndDerivatives=provide  SimscapeFilterOrder=1  InputFilterTimeConstant=0.001  UdotUserProvided=0
  Voltage Sensor : fl_lib/Electrical/Electrical Sensors/Voltage Sensor
  In : PMIOPort  Side=Left
  ~ : PMIOPort  Port=2  Side=Right
  Vdc : Outport
  wires:
  Grid_ref/1 -> Simulink-PS Converter4/1
  Chopper/1 -> Scope/1, Simulink-PS Converter2/1
  PS-Simulink Converter1/1 -> Vdc/1  "Vdc"
  SM_ref/1 -> Simulink-PS Converter/1
  connections:
  Electrical Reference/LConn1 -- Machine Side Converter/RConn2 -- Voltage Sensor/RConn2 -- Capacitor/RConn1
  Grid Side Converter/RConn1 -- Ideal Semiconductor Switch/RConn1 -- Capacitor/LConn1 -- Machine Side Converter/RConn1 -- Voltage Sensor/LConn1
  Electrical Reference2/LConn1 -- Grid Side Converter/RConn2
  PS-Simulink Converter1/LConn1 -- Voltage Sensor/RConn1
  ~/RConn1 -- Grid Side Converter/LConn2
  Resistor/LConn1 -- Ideal Semiconductor Switch/RConn2
  Grid Side Converter/LConn1 -- Simulink-PS Converter4/RConn1
  Electrical Reference1/LConn1 -- Resistor/RConn1
  Simulink-PS Converter2/RConn1 -- Ideal Semiconductor Switch/LConn1
  Machine Side Converter/LConn2 -- In/RConn1
  Simulink-PS Converter/RConn1 -- Machine Side Converter/LConn1

== system SimscapeCustomComponents_lib/Microgrid and Renewables/Sources/Wind Plant/Back-to-Back Converters/Switching ==
  Chopper : Inport
  SM_ref : Inport  Port=2
  Grid_ref : Inport  Port=3
  Capacitor : fl_lib/Electrical/Electrical Elements/Capacitor  c=capacitance F  r=1e-1 Ohm  g=0 1/Ohm  i_specify=off  i_priority=None  i=0 A  i_nominal_specify=off  i_nominal_value=1  i_nominal_unit=A  v_specify=off  v_priority=None  v=0 V  v_nominal_specify=off  v_nominal_value=1  v_nominal_unit=V  vc_specify=on  vc_priority=High  vc=baseVoltageDC V  vc_nominal_specify=off  vc_nominal_value=1  vc_nominal_unit=V
  Electrical Reference : fl_lib/Electrical/Electrical Elements/Electrical Reference
  Electrical Reference1 : fl_lib/Electrical/Electrical Elements/Electrical Reference
  Electrical Reference2 : fl_lib/Electrical/Electrical Elements/Electrical Reference
  Grid Side Converter : Subsystem
      settings: PortSchema="{\"entries\":[{\"content\":{\"sides\":[{\"content\":{\"connectorIds\":[\"LConn1\",\"LConn2\"]},\"type\":\"ConnectorPlacement.EquallySpacedRectSide\",\"uuid\":\"e32be008-cebd-46aa-ba62-c5c92b9b23e3\"},{\"content\":{\"connectorIds\":[\"In1\",\"RConn1\"],\"side\":\"RIGHT\"},\"type\":\"ConnectorPlacement.EquallySpacedRectSide\",\"uuid\":\"c483e451-04b5-4212-bdd1-c589ba5bea78\"},{\"content\":{\"side\":\"TOP\"},\"type\":\"ConnectorPlacement.EquallySpacedRectSide\",\"uuid\":\"824c135c-7e5f-4da0-a7de-e626b4bfa50d\"}]},\"type\":\"ConnectorPlacement.EquallySpacedConnector\",\"uuid\":\"5f81c72d-92ab-4525-91a6-193f769a7c86\"}],\"packageUris\":[\"http://schema.mathworks.com/mf0/Connector/R2020b\"],\"version\":\"1.0\"}"
  Ideal Semiconductor Switch : ee_lib/Semiconductors & Converters/Ideal Semiconductor Switch  port_option=ee.enum.controlport.ps  Ron=0.001 Ohm  Goff=1e-6 1/Ohm  Vth=0.5 V  diode_param=ee.enum.converters.protectiondiode.none  diode_Vf=0.8 V  diode_Ron=0.001 Ohm  diode_Goff=1e-5 1/Ohm  diode_C=50e-9 F  diode_iRM=-235 A  diode_iF=300 A  diode_idot=-50 A/us  diode_trr_param=ee.enum.converters.diodetrr.trr_factor  diode_trr_factor=3  diode_trr=15 us  diode_Qrr=1500 s*uA
  Machine Side Converter : Subsystem
      settings: PortSchema="{\"entries\":[{\"content\":{\"sides\":[{\"content\":{\"connectorIds\":[\"LConn1\",\"LConn2\"]},\"type\":\"ConnectorPlacement.EquallySpacedRectSide\",\"uuid\":\"e32be008-cebd-46aa-ba62-c5c92b9b23e3\"},{\"content\":{\"connectorIds\":[\"In1\",\"RConn1\"],\"side\":\"RIGHT\"},\"type\":\"ConnectorPlacement.EquallySpacedRectSide\",\"uuid\":\"c483e451-04b5-4212-bdd1-c589ba5bea78\"},{\"content\":{\"side\":\"TOP\"},\"type\":\"ConnectorPlacement.EquallySpacedRectSide\",\"uuid\":\"824c135c-7e5f-4da0-a7de-e626b4bfa50d\"}]},\"type\":\"ConnectorPlacement.EquallySpacedConnector\",\"uuid\":\"5f81c72d-92ab-4525-91a6-193f769a7c86\"}],\"packageUris\":[\"http://schema.mathworks.com/mf0/Connector/R2020b\"],\"version\":\"1.0\"}"
  PS-Simulink Converter1 : nesl_utility/PS-Simulink Converter  PhysicalDomain=network_engine_domain  SubClassName=ps_output  LeftPortType=input  RightPortType=output  PseudoPeriodic=off  Frequencies=[]  VectorFormat=1-D array  Unit=V  AffineConversion=off
  Resistor : fl_lib/Electrical/Electrical Elements/Resistor  R=16 Ohm  i_specify=off  i_priority=None  i=0 A  i_nominal_specify=off  i_nominal_value=1  i_nominal_unit=A  v_specify=off  v_priority=None  v=0 V  v_nominal_specify=off  v_nominal_value=1  v_nominal_unit=V
  Scope : Scope
      settings: ActiveDisplayYMinimum=-0.125  ActiveDisplayYMaximum=1.125  DataLoggingVariableName=ScopeData11
  Simulink-PS Converter2 : nesl_utility/Simulink-PS Converter  PhysicalDomain=network_engine_domain  SubClassName=ps_input  LeftPortType=input  RightPortType=output  PseudoPeriodic=off  Frequencies=[]  NoiseDistribution=none  NoiseParameters=[]  Unit=1  AffineConversion=off  FilteringAndDerivatives=provide  SimscapeFilterOrder=1  InputFilterTimeConstant=0.001  UdotUserProvided=0
  Voltage Sensor : fl_lib/Electrical/Electrical Sensors/Voltage Sensor
  In : PMIOPort  Side=Left
  ~ : PMIOPort  Port=2  Side=Right
  Vdc : Outport
  wires:
  SM_ref/1 -> Machine Side Converter/1(mabc)
  Grid_ref/1 -> Grid Side Converter/1(mabc)
  Chopper/1 -> Scope/1, Simulink-PS Converter2/1
  PS-Simulink Converter1/1 -> Vdc/1  "Vdc"
  connections:
  Machine Side Converter/LConn2 -- Voltage Sensor/RConn2 -- Capacitor/RConn1 -- Electrical Reference/LConn1
  Ideal Semiconductor Switch/RConn1 -- Grid Side Converter/LConn1 -- Capacitor/LConn1 -- Machine Side Converter/LConn1 -- Voltage Sensor/LConn1
  Grid Side Converter/LConn2 -- Electrical Reference2/LConn1
  PS-Simulink Converter1/LConn1 -- Voltage Sensor/RConn1
  ~/RConn1 -- Grid Side Converter/RConn1
  Resistor/LConn1 -- Ideal Semiconductor Switch/RConn2
  Electrical Reference1/LConn1 -- Resistor/RConn1
  Simulink-PS Converter2/RConn1 -- Ideal Semiconductor Switch/LConn1
  Machine Side Converter/RConn1 -- In/RConn1
